simulink model "cic_int_sim"  (R2023a)
settings: Solver=VariableStepAuto  StartTime=0.0  StopTime=t  RelTol=1e-3
InitFcn:
  | initial_par
undefined symbols (not defined in the file): cp2, fin1, fs, hb1, N, utest
libraries: dspsigops x5, SDtoolbox x4, spspowerguiLib x1
settings Model: Creator=LZD  LastModifiedBy=86198
settings DataIOCC: ReturnWorkspaceOutputs=off
settings DebuggingCC: UnconnectedInputMsg=warning  UnconnectedOutputMsg=warning  UnconnectedLineMsg=warning
settings ModelReferenceCC: EnableRefExpFcnMdlSchedulingChecks=on
settings RTWCC: DLArmComputeVersion=19.05

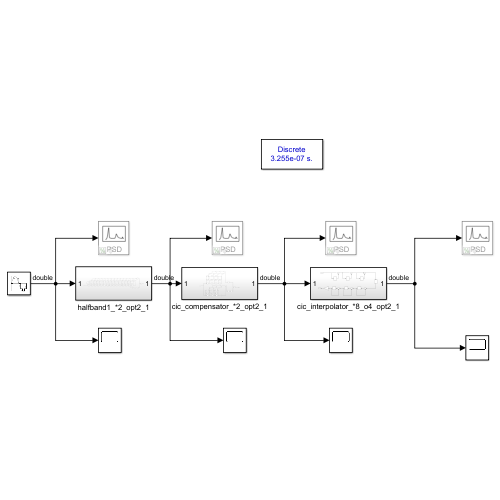
[thumbnail: Simulink's stored preview of the top-level diagram]
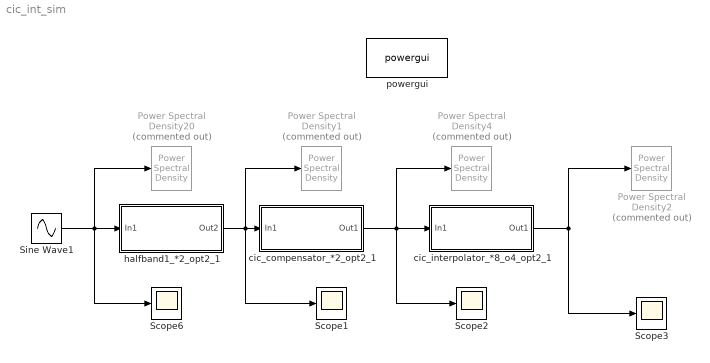
== system cic_int_sim ==
  Power Spectral Density1 : SDtoolbox/Power Spectral Density  Commented=on  SN=2  Fs=fs*2  fBL=20  fBH=20e3  Fin=fin1  N=N  Ntransient=Ntransient  VW=on  savename=savemat  Scale_type=linear
      settings: SourceProductName=SDtoolbox
  Power Spectral Density2 : SDtoolbox/Power Spectral Density  Commented=on  SN=4  Fs=fs*64  fBL=20  fBH=20e3  Fin=fin1  N=N  Ntransient=Ntransient  VW=on  savename=savemat  Scale_type=linear
      settings: SourceProductName=SDtoolbox
  Power Spectral Density20 : SDtoolbox/Power Spectral Density  Commented=on  SN=1  Fs=fs  fBL=20  fBH=20e3  Fin=fin1  N=N  Ntransient=Ntransient  VW=on  savename=savemat  Scale_type=linear
      settings: SourceProductName=SDtoolbox
  Power Spectral Density4 : SDtoolbox/Power Spectral Density  Commented=on  SN=3  Fs=fs*2*2  fBL=20  fBH=20e3  Fin=fin1  N=N  Ntransient=Ntransient  VW=on  savename=savemat  Scale_type=linear
      settings: SourceProductName=SDtoolbox
  Scope{1..3,6} (4 alike) : Scope
  Sine Wave1 : Sin  Amplitude=utest  Frequency=2*pi*fin1  SampleTime=1/fs
  cic_compensator_*2_opt2_1 : Subsystem
  cic_interpolator_*8_o4_opt2_1 : Subsystem
  halfband1_*2_opt2_1 : Subsystem
  powergui : spspowerguiLib/powergui  Priority=1  SimulationMode=Discrete  SampleTime=1/fs/64  frequency=60  Iterations=50  frequencyindice=60  Pbase=100e6  ErrMax=1e-4  UnitsV=kV  UnitsW=MW  buscounter=0  FunctionMessages=off  echomessages=off  EnableUseOfTLC=off  CurrentSourceSwitches=off  DisableSnubberDevices=off  DisableRonSwitches=off  DisableVfSwitches=off  DisplayEquations=off  AutomaticDiscreteSolvers=off  SolverType=Tustin/Backward Euler (TBE)  Interpol=off  ExternalGateDelay=off  methode=off  Ts=100  x0status=blocks  SPID=on  SwTol=0  HookPort=off  NonlinearTolerance=1e-4  nMaxIteration=100  ContinueOnMaxIteration=off  RestoreLinks=warning  ResistiveCurrentMeasurement=off  Frange=[0:2:500]  Ylog=off  Xlog=on  ShowGrid=off  save=off  variable=ZData  structure=0  ZoomFFT=off  StartTime=0.0  cycles=1  DisplayStyle=1  fundamental=60  FreqAxis=off  MaxFrequency=1000  frequencyindicesteady=1  RmsSteady=1  display=off
  wires:
  Sine Wave1/1 -> halfband1_*2_opt2_1/1(In1), Scope6/1, Power Spectral Density20/1
  cic_compensator_*2_opt2_1/1(Out1) -> cic_interpolator_*8_o4_opt2_1/1(In1), Scope2/1, Power Spectral Density4/1
  cic_interpolator_*8_o4_opt2_1/1(Out1) -> Scope3/1, Power Spectral Density2/1
  halfband1_*2_opt2_1/1(Out2) -> cic_compensator_*2_opt2_1/1(In1), Power Spectral Density1/1, Scope1/1

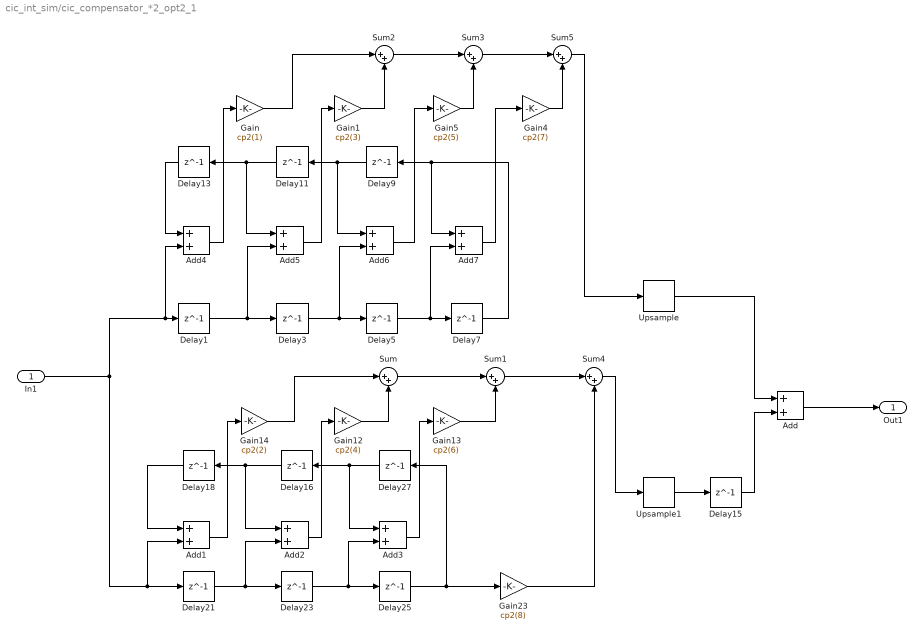
== system cic_int_sim/cic_compensator_*2_opt2_1 ==
  In1 : Inport
  Add{,1..7} (8 alike) : Sum
  Delay{1,3,5,7,9,11,13,15..16,18,21,23,25,27} (14 alike) : Delay  DelayLength=1  InitialCondition=0
  Gain : Gain  Gain=cp2(1)
  Gain1 : Gain  Gain=cp2(3)
  Gain12 : Gain  Gain=cp2(4)
  Gain13 : Gain  Gain=cp2(6)
  Gain14 : Gain  Gain=cp2(2)
  Gain23 : Gain  Gain=cp2(8)
  Gain4 : Gain  Gain=cp2(7)
  Gain5 : Gain  Gain=cp2(5)
  Sum{,1..5} (6 alike) : Sum  Inputs=|++
  Upsample : dspsigops/Upsample  FactorSource=Dialog parameter  N=2  Nmax=16  phase=0  RateOptions=Allow multirate processing  ic=0  mode=Unused parameter value
  Upsample1 : dspsigops/Upsample  FactorSource=Dialog parameter  N=2  Nmax=16  phase=0  RateOptions=Allow multirate processing  ic=0  mode=Unused parameter value
  Out1 : Outport
  wires:
  Delay1/1 -> Add5/2, Delay3/1
  Delay5/1 -> Add7/2, Delay7/1
  Delay3/1 -> Add6/2, Delay5/1
  Delay11/1 -> Add5/1, Delay13/1
  Delay9/1 -> Add6/1, Delay11/1
  Delay25/1 -> Delay27/1, Gain23/1
  Delay18/1 -> Add1/1
  Delay23/1 -> Add3/2, Delay25/1
  Delay21/1 -> Add2/2, Delay23/1
  Delay16/1 -> Add2/1, Delay18/1
  Delay27/1 -> Delay16/1, Add3/1
  In1/1 -> Add4/2, Delay1/1, Add1/2, Delay21/1
  Upsample1/1 -> Delay15/1
  Add/1 -> Out1/1
  Upsample/1 -> Add/1
  Delay15/1 -> Add/2
  Add1/1 -> Gain14/1
  Add2/1 -> Gain12/1
  Add3/1 -> Gain13/1
  Gain14/1 -> Sum/1
  Gain12/1 -> Sum/2
  Sum/1 -> Sum1/1
  Gain13/1 -> Sum1/2
  Sum1/1 -> Sum4/1
  Gain23/1 -> Sum4/2
  Sum4/1 -> Upsample1/1
  Delay13/1 -> Add4/1
  Add4/1 -> Gain/1
  Delay7/1 -> Add7/1, Delay9/1
  Add5/1 -> Gain1/1
  Add6/1 -> Gain5/1
  Add7/1 -> Gain4/1
  Gain/1 -> Sum2/1
  Gain1/1 -> Sum2/2
  Gain5/1 -> Sum3/2
  Sum2/1 -> Sum3/1
  Sum3/1 -> Sum5/1
  Gain4/1 -> Sum5/2
  Sum5/1 -> Upsample/1

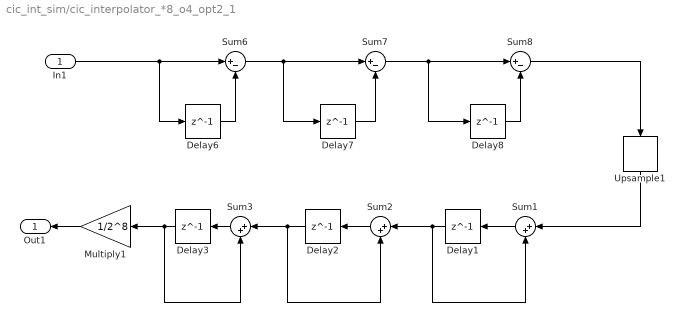
== system cic_int_sim/cic_interpolator_*8_o4_opt2_1 ==
  In1 : Inport
  Delay{1..3,6..8} (6 alike) : Delay  DelayLength=1  InitialCondition=0
  Multiply1 : Gain  Gain=1/2^8
  Sum1 : Sum  Inputs=|++
  Sum2 : Sum  Inputs=|++
  Sum3 : Sum  Inputs=|++
  Sum6 : Sum  Inputs=|+-
  Sum7 : Sum  Inputs=|+-
  Sum8 : Sum  Inputs=|+-
  Upsample1 : dspsigops/Upsample  FactorSource=Dialog parameter  N=8  Nmax=16  phase=0  RateOptions=Allow multirate processing  ic=0  mode=Unused parameter value
  Out1 : Outport
  wires:
  Delay6/1 -> Sum6/2
  Delay2/1 -> Sum3/1, Sum2/2
  Delay8/1 -> Sum8/2
  Delay7/1 -> Sum7/2
  Sum7/1 -> Delay8/1, Sum8/1
  Delay1/1 -> Sum2/1, Sum1/2
  Sum6/1 -> Delay7/1, Sum7/1
  In1/1 -> Sum6/1, Delay6/1
  Multiply1/1 -> Out1/1
  Sum3/1 -> Delay3/1
  Delay3/1 -> Sum3/2, Multiply1/1
  Sum2/1 -> Delay2/1
  Sum1/1 -> Delay1/1
  Upsample1/1 -> Sum1/1
  Sum8/1 -> Upsample1/1

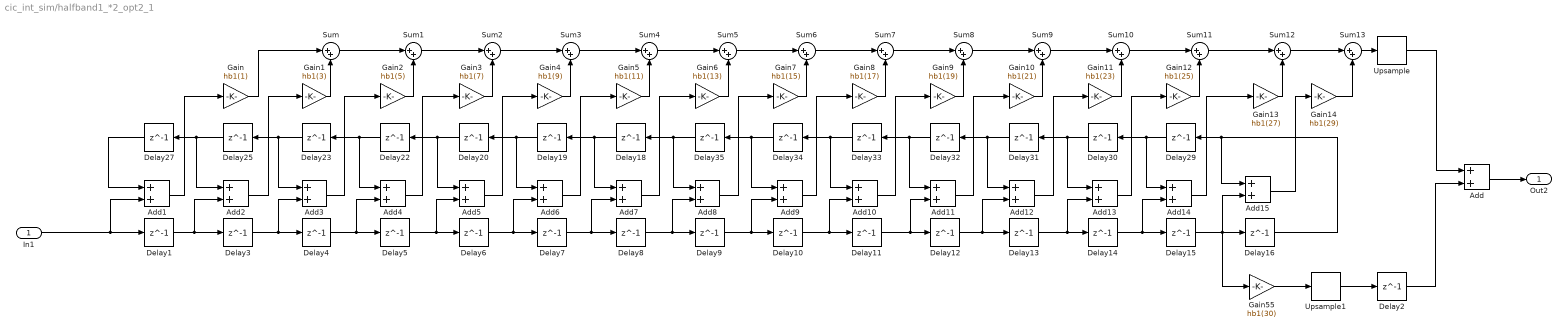
== system cic_int_sim/halfband1_*2_opt2_1 ==
  In1 : Inport
  Add{,1..15} (16 alike) : Sum
  Delay{1..16,18..20,22..23,25,27,29..35} (30 alike) : Delay  DelayLength=1  InitialCondition=0
  Gain : Gain  Gain=hb1(1)
  Gain1 : Gain  Gain=hb1(3)
  Gain10 : Gain  Gain=hb1(21)
  Gain11 : Gain  Gain=hb1(23)
  Gain12 : Gain  Gain=hb1(25)
  Gain13 : Gain  Gain=hb1(27)
  Gain14 : Gain  Gain=hb1(29)
  Gain2 : Gain  Gain=hb1(5)
  Gain3 : Gain  Gain=hb1(7)
  Gain4 : Gain  Gain=hb1(9)
  Gain5 : Gain  Gain=hb1(11)
  Gain55 : Gain  Gain=hb1(30)
  Gain6 : Gain  Gain=hb1(13)
  Gain7 : Gain  Gain=hb1(15)
  Gain8 : Gain  Gain=hb1(17)
  Gain9 : Gain  Gain=hb1(19)
  Sum{,1..13} (14 alike) : Sum  Inputs=|++
  Upsample : dspsigops/Upsample  FactorSource=Dialog parameter  N=2  Nmax=16  phase=0  RateOptions=Allow multirate processing  ic=0  mode=Unused parameter value
  Upsample1 : dspsigops/Upsample  FactorSource=Dialog parameter  N=2  Nmax=16  phase=0  RateOptions=Allow multirate processing  ic=0  mode=Unused parameter value
  Out2 : Outport
  wires:
  Add/1 -> Out2/1
  Upsample/1 -> Add/1
  In1/1 -> Delay1/1, Add1/2
  Upsample1/1 -> Delay2/1
  Delay2/1 -> Add/2
  Gain55/1 -> Upsample1/1
  Add1/1 -> Gain/1
  Add2/1 -> Gain1/1
  Delay1/1 -> Add2/2, Delay3/1
  Delay3/1 -> Add3/2, Delay4/1
  Add3/1 -> Gain2/1
  Delay4/1 -> Add4/2, Delay5/1
  Add4/1 -> Gain3/1
  Delay5/1 -> Add5/2, Delay6/1
  Add5/1 -> Gain4/1
  Delay6/1 -> Add6/2, Delay7/1
  Add6/1 -> Gain5/1
  Delay7/1 -> Add7/2, Delay8/1
  Add7/1 -> Gain6/1
  Delay8/1 -> Add8/2, Delay9/1
  Add8/1 -> Gain7/1
  Delay9/1 -> Add9/2, Delay10/1
  Add9/1 -> Gain8/1
  Delay10/1 -> Add10/2, Delay11/1
  Add10/1 -> Gain9/1
  Delay11/1 -> Add11/2, Delay12/1
  Add11/1 -> Gain10/1
  Delay12/1 -> Add12/2, Delay13/1
  Add12/1 -> Gain11/1
  Delay13/1 -> Add13/2, Delay14/1
  Add13/1 -> Gain12/1
  Delay14/1 -> Add14/2, Delay15/1
  Add14/1 -> Gain13/1
  Delay15/1 -> Gain55/1, Delay16/1, Add15/2
  Delay19/1 -> Add6/1, Delay20/1
  Delay29/1 -> Add14/1, Delay30/1
  Delay34/1 -> Delay35/1, Add9/1
  Delay18/1 -> Add7/1, Delay19/1
  Delay20/1 -> Add5/1, Delay22/1
  Delay33/1 -> Delay34/1, Add10/1
  Delay22/1 -> Add4/1, Delay23/1
  Delay32/1 -> Add11/1, Delay33/1
  Delay35/1 -> Add8/1, Delay18/1
  Delay23/1 -> Delay25/1, Add3/1
  Delay30/1 -> Add13/1, Delay31/1
  Delay31/1 -> Add12/1, Delay32/1
  Delay25/1 -> Add2/1, Delay27/1
  Delay27/1 -> Add1/1
  Gain1/1 -> Sum/2
  Gain/1 -> Sum/1
  Sum/1 -> Sum1/1
  Gain2/1 -> Sum1/2
  Sum1/1 -> Sum2/1
  Gain3/1 -> Sum2/2
  Sum2/1 -> Sum3/1
  Gain4/1 -> Sum3/2
  Sum3/1 -> Sum4/1
  Gain5/1 -> Sum4/2
  Sum4/1 -> Sum5/1
  Gain6/1 -> Sum5/2
  Gain7/1 -> Sum6/2
  Sum5/1 -> Sum6/1
  Sum6/1 -> Sum7/1
  Gain8/1 -> Sum7/2
  Sum7/1 -> Sum8/1
  Gain9/1 -> Sum8/2
  Sum8/1 -> Sum9/1
  Gain10/1 -> Sum9/2
  Sum9/1 -> Sum10/1
  Gain11/1 -> Sum10/2
  Sum10/1 -> Sum11/1
  Gain12/1 -> Sum11/2
  Sum11/1 -> Sum12/1
  Gain13/1 -> Sum12/2
  Sum12/1 -> Sum13/1
  Gain14/1 -> Sum13/2
  Sum13/1 -> Upsample/1
  Delay16/1 -> Add15/1, Delay29/1
  Add15/1 -> Gain14/1
